simulink library "LumControlsBlockset"  (R2018b)
settings: Solver=ode45  StartTime=0.0  StopTime=10.0  RelTol=1e-3  EnableMultiTasking=on
undefined symbols (not defined in the file): A, B, C, D, L, T, xhat_0
settings Model: Creator=Christopher  LastModifiedBy=Christopher
settings DataIOCC: LimitDataPoints=on  SaveFormat=Array
settings OptimizationCC: LifeSpan=inf
settings DebuggingCC: SolverPrmCheckMsg=warning  SFUnexpectedBacktrackingDiag=warning  SFNoUnconditionalDefaultTransitionDiag=warning  SFExecutionAtInitializationDiag=none
settings HardwareCC: ProdBitPerPointer=32  ProdBitPerSizeT=32  ProdBitPerPtrDiffT=32  ProdLargestAtomicFloat=None  ProdIntDivRoundTo=Undefined  ProdEndianess=Unspecified  ProdWordSize=32  ProdHWDeviceType=32-bit Generic
settings ModelReferenceCC: PropagateSignalLabelsOutOfModel=off
settings SFSimCC: SimUseLocalCustomCode=off
settings RTWCC: RTWUseLocalCustomCode=off
settings CodeAppCC: StateflowObjectComments=on
settings GRTTargetCC: TargetLangStandard=C89/C90 (ANSI)  GeneratePreprocessorConditionals=Disable all
settings ConfigComp: CovMetricSettings=dw  CovHtmlReporting=on  CovSaveCumulativeToWorkspaceVar=on  CovSaveSingleToWorkspaceVar=on  CovExternalEMLEnable=off  CovSFcnEnable=off

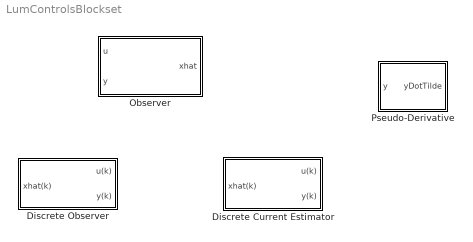
== system LumControlsBlockset ==
  Discrete Current Estimator : Subsystem
  Discrete Observer : Subsystem  mask{A=A, B=B, C=C, D=D, L=L, xhat_0=xhat_0, T=T}
      mask prompts: A "A (A matrix)"; B "B (B matrix)"; C "C (C matrix)"; D "D (D matrix)"; L "L (Kalman Gain)"; xhat_0 "xhat(0) (Initial Condition)"; T "T (Sampling Time)"
      mask help:
      | Implement a Kalman filter estimator.  Dynamics goverened by
      |
      | 	xhat(k+1) = A*xhat(k) + B*u(k) + L[y(k) - yhat(k)]
      |
      | where	yhat(k) = C*xhat(k) + D*u(k)
      |
      | Dynamics of this system should be governed by eig(A-L*C)
      |
      | Created by Christopher Lum
      | lum@u.washington.edu
  Observer : Subsystem  mask{A=0, B=0, C=0, D=0, L=0, xhat0=0}
      mask prompts: L "L (observer gain)"; xhat0 "Initial condition of observer (xhat0)"
      mask help:
      | Implement a standard, continuous, linear observer with dynamics of
      |
      | xhatDot = A*xhat + B*u + L(y - yhat)
      |
      | where yhat = C*xhat + D*u
  Pseudo-Derivative : Subsystem  mask{a=0}
      mask prompts: a "Break frequency (rad/s)"
      mask help:
      | A simple pseudo-derivative implemented as a transfer function of
      |
      |               a*s
      | G(s) = -------
      |              s + a
      |
      | PARAMETERS:
      | a = break frequency of low-pass filter component of pseudo-derivative
      |
      | INPUT:
      | y = input signal
      |
      | OUTPUT:
      | yDotTilde = approximate derivative of y
      |
      | Created by Christopher Lum
      | lum@uw.edu

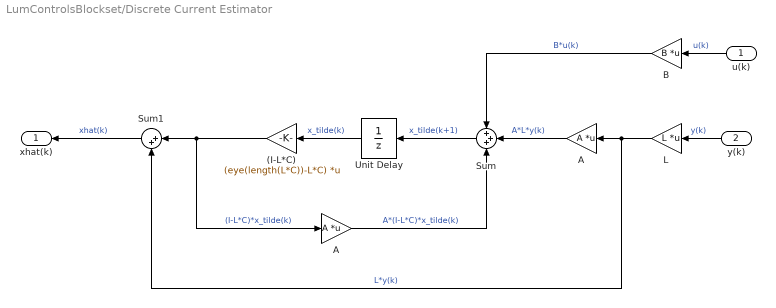
== system LumControlsBlockset/Discrete Current Estimator ==
  u(k) : Inport
  y(k) : Inport  Port=2
  (I-L*C) : Gain  Gain=(eye(length(L*C))-L*C)  Multiplication=Matrix(K*u)  SaturateOnIntegerOverflow=on  OutDataTypeStr=Inherit: Same as input  ParamDataTypeStr=Inherit: Same as input
  A : Gain  Gain=A  Multiplication=Matrix(K*u)  SaturateOnIntegerOverflow=on  OutDataTypeStr=Inherit: Same as input  ParamDataTypeStr=Inherit: Same as input
  "A " : Gain  Gain=A  Multiplication=Matrix(K*u)  SaturateOnIntegerOverflow=on  OutDataTypeStr=Inherit: Same as input  ParamDataTypeStr=Inherit: Same as input
  B : Gain  Gain=B  Multiplication=Matrix(K*u)  SaturateOnIntegerOverflow=on  OutDataTypeStr=Inherit: Same as input  ParamDataTypeStr=Inherit: Same as input
  L : Gain  Gain=L  Multiplication=Matrix(K*u)  SaturateOnIntegerOverflow=on  OutDataTypeStr=Inherit: Same as input  ParamDataTypeStr=Inherit: Same as input
  Sum : Sum  Inputs=+++  SaturateOnIntegerOverflow=on
  Sum1 : Sum  Inputs=|++  SaturateOnIntegerOverflow=on
  Unit Delay : UnitDelay  SampleTime=T
  xhat(k) : Outport
  wires:
  Sum/1 -> Unit Delay/1  "x_tilde(k+1)"
  Unit Delay/1 -> (I-L*C)/1  "x_tilde(k)"
  y(k)/1 -> L/1  "y(k)"
  u(k)/1 -> B/1  "u(k)"
  B/1 -> Sum/1  "B*u(k)"
  L/1 -> "A "/1, Sum1/2  "L*y(k)"
  A/1 -> Sum/3  "A*(I-L*C)*x_tilde(k)"
  (I-L*C)/1 -> A/1, Sum1/1  "(I-L*C)*x_tilde(k)"
  "A "/1 -> Sum/2  "A*L*y(k)"
  Sum1/1 -> xhat(k)/1  "xhat(k)"

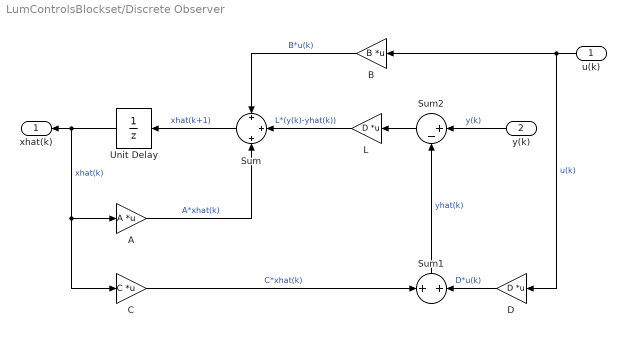
== system LumControlsBlockset/Discrete Observer ==
  u(k) : Inport
  y(k) : Inport  Port=2
  A : Gain  Gain=A  Multiplication=Matrix(K*u)  SaturateOnIntegerOverflow=on  OutDataTypeStr=Inherit: Same as input  ParamDataTypeStr=Inherit: Same as input
  B : Gain  Gain=B  Multiplication=Matrix(K*u)  SaturateOnIntegerOverflow=on  OutDataTypeStr=Inherit: Same as input  ParamDataTypeStr=Inherit: Same as input
  C : Gain  Gain=C  Multiplication=Matrix(K*u)  SaturateOnIntegerOverflow=on  OutDataTypeStr=Inherit: Same as input  ParamDataTypeStr=Inherit: Same as input
  D : Gain  Gain=D  Multiplication=Matrix(K*u)  SaturateOnIntegerOverflow=on  OutDataTypeStr=Inherit: Same as input  ParamDataTypeStr=Inherit: Same as input
  L : Gain  Gain=D  Multiplication=Matrix(K*u)  SaturateOnIntegerOverflow=on  OutDataTypeStr=Inherit: Same as input  ParamDataTypeStr=Inherit: Same as input
  Sum : Sum  Inputs=+|+|+  SaturateOnIntegerOverflow=on
  Sum1 : Sum  Inputs=+|+  SaturateOnIntegerOverflow=on
  Sum2 : Sum  Inputs=|+-  SaturateOnIntegerOverflow=on
  Unit Delay : UnitDelay  InitialCondition=xhat_0  SampleTime=T
  xhat(k) : Outport
  wires:
  y(k)/1 -> Sum2/1  "y(k)"
  Sum2/1 -> L/1
  Sum1/1 -> Sum2/2  "yhat(k)"
  D/1 -> Sum1/2  "D*u(k)"
  C/1 -> Sum1/1  "C*xhat(k)"
  L/1 -> Sum/2  "L*(y(k)-yhat(k))"
  B/1 -> Sum/1  "B*u(k)"
  A/1 -> Sum/3  "A*xhat(k)"
  Sum/1 -> Unit Delay/1  "xhat(k+1)"
  u(k)/1 -> D/1, B/1  "u(k)"
  Unit Delay/1 -> xhat(k)/1, C/1, A/1  "xhat(k)"

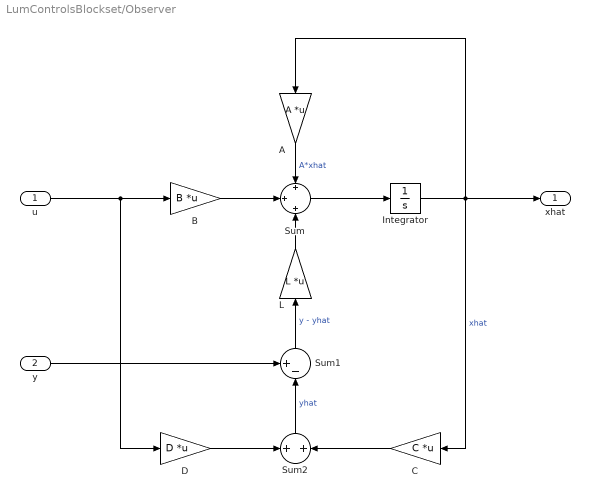
== system LumControlsBlockset/Observer ==
  u : Inport
  y : Inport  Port=2
  A : Gain  Gain=A  Multiplication=Matrix(K*u)
  B : Gain  Gain=B  Multiplication=Matrix(K*u)
  C : Gain  Gain=C  Multiplication=Matrix(K*u)
  D : Gain  Gain=D  Multiplication=Matrix(K*u)
  Integrator : Integrator  InitialCondition=xhat0
  L : Gain  Gain=L  Multiplication=Matrix(K*u)
  Sum : Sum  Inputs=+|+|+
  Sum1 : Sum  Inputs=+-|
  Sum2 : Sum  Inputs=+|+
  xhat : Outport
  wires:
  Sum2/1 -> Sum1/2  "yhat"
  Sum1/1 -> L/1  "y - yhat"
  y/1 -> Sum1/1
  C/1 -> Sum2/2
  D/1 -> Sum2/1
  u/1 -> D/1, B/1
  L/1 -> Sum/3
  Integrator/1 -> C/1, A/1, xhat/1  "xhat"
  A/1 -> Sum/1  "A*xhat"
  B/1 -> Sum/2
  Sum/1 -> Integrator/1

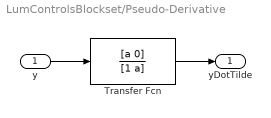
== system LumControlsBlockset/Pseudo-Derivative ==
  y : Inport
  Transfer Fcn : TransferFcn  Numerator=[a 0]  Denominator=[1 a]
  yDotTilde : Outport
  wires:
  y/1 -> Transfer Fcn/1
  Transfer Fcn/1 -> yDotTilde/1
